simulink model "start_process"  (R2019a)
settings: Solver=FixedStepAuto  StartTime=0.0  StopTime=0.001  RelTol=1e-3
values from neighbouring files (symbols this model uses):
  trigger = true    [final_test.m]    (also in main_file.m; vel_measurement_final.m)
  v_m = 0.5*median(vel_norm(end-4:end)) + 0.5*mean(vel_norm(end-4:end))    [final_test.m]    (also in main_file.m = mean(vel_norm(end-3:end)) * 1000; vel_measurement_final.m = mean(vel_norm(end-3:end)); vel_test_25_3_2019.m = mean(vel_norm(end-3:end)))
libraries: TcAdsLib x3
settings Model: Creator=chijiang  LastModifiedBy=chijiang
settings DataIOCC: ReturnWorkspaceOutputs=off
settings OptimizationCC: LocalBlockOutputs=off
settings DebuggingCC: ArithmeticOperatorsInVariantConditions=warning
settings RTWCC: SystemTargetFile=TwinCAT.tlc  MakeCommand=make_tct  TemplateMakefile=tct_msbuild.tmf  Description=TwinCAT Target  GenerateReport=on  TargetLang=C++
settings STFCustomTargetCC: TargetLangStandard=C++03 (ISO)  CompOptLevelCompliant=on  MATLABClassNameForMDSCustomization=Simulink.SoftwareTarget.TargetSpecificTriggerConfigurationBase  SystemTargetFile=TwinCAT.tlc

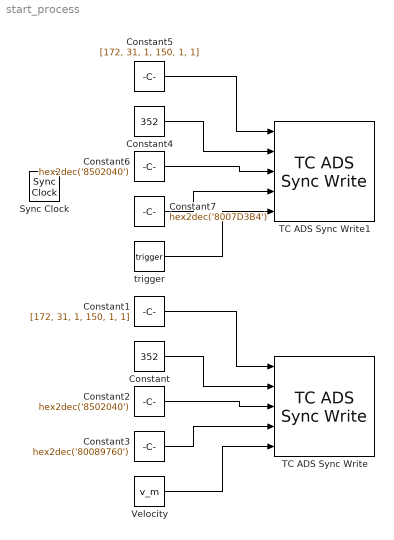
== system start_process ==
  Constant : Constant  Value=352  OutDataTypeStr=uint16
  Constant1 : Constant  Value=[172, 31, 1, 150, 1, 1]  OutDataTypeStr=uint8
  Constant2 : Constant  Value=hex2dec('8502040')  OutDataTypeStr=uint32
  Constant3 : Constant  Value=hex2dec('80089760')  OutDataTypeStr=uint32
  Constant4 : Constant  Value=352  OutDataTypeStr=uint16
  Constant5 : Constant  Value=[172, 31, 1, 150, 1, 1]  OutDataTypeStr=uint8
  Constant6 : Constant  Value=hex2dec('8502040')  OutDataTypeStr=uint32
  Constant7 : Constant  Value=hex2dec('8007D3B4')  OutDataTypeStr=uint32
  Sync Clock : TcAdsLib/Utilities/Sync Clock  OutputPortSelect=None  InputPortSelect=None
      settings: SourceProductName=Beckhoff TwinCAT ADS Interface
  TC ADS Sync Write : TcAdsLib/Synchronous/TC ADS Sync Write  SampleTime=-1  AbortSimulationOnAdsError=off  WriteDataType=double  WriteDataDim=1  WriteDataColToRowMajor=on  AdsTimeout=1  DirectFeedThrough=off  CreateSignalLabels=on  CodeGenConnectType=DataArea (OutputSrc)
      settings: SourceProductName=Beckhoff TwinCAT ADS Interface
  TC ADS Sync Write1 : TcAdsLib/Synchronous/TC ADS Sync Write  SampleTime=-1  AbortSimulationOnAdsError=off  WriteDataType=double  WriteDataDim=1  WriteDataColToRowMajor=on  AdsTimeout=1  DirectFeedThrough=off  CreateSignalLabels=on  CodeGenConnectType=DataArea (OutputSrc)
      settings: SourceProductName=Beckhoff TwinCAT ADS Interface
  Velocity : Constant  Value=v_m
  trigger : Constant  Value=trigger  OutDataTypeStr=double
  wires:
  Constant/1 -> TC ADS Sync Write/2
  Velocity/1 -> TC ADS Sync Write/5
  Constant1/1 -> TC ADS Sync Write/1
  Constant2/1 -> TC ADS Sync Write/3
  Constant3/1 -> TC ADS Sync Write/4
  Constant7/1 -> TC ADS Sync Write1/4
  Constant6/1 -> TC ADS Sync Write1/3
  Constant5/1 -> TC ADS Sync Write1/1
  trigger/1 -> TC ADS Sync Write1/5
  Constant4/1 -> TC ADS Sync Write1/2
